simulink library "csc_ln200_lib_a"  (R2014b)
settings: Solver=ode45  SolverMode=SingleTasking  StartTime=0.0  StopTime=10.0  RelTol=1e-3
undefined symbols (not defined in the file or in its folder): est_time_step, sim_time_step_size
libraries: simulink x3, util_common_lib x2, csc_ln200_lib_a x2, util_info_lib x1, csu_imk_imu_kinematics_lib_a x1, csu_lnh_ln200_hardware_lib_a x1
settings Model: Creator=hcannon  LastModifiedBy=mstewart

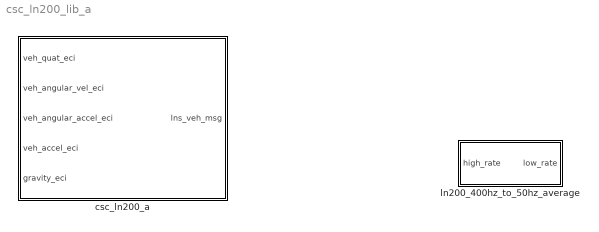
== system csc_ln200_lib_a ==
  csc_ln200_a : Subsystem
  ln200_400hz_to_50hz_average : Subsystem

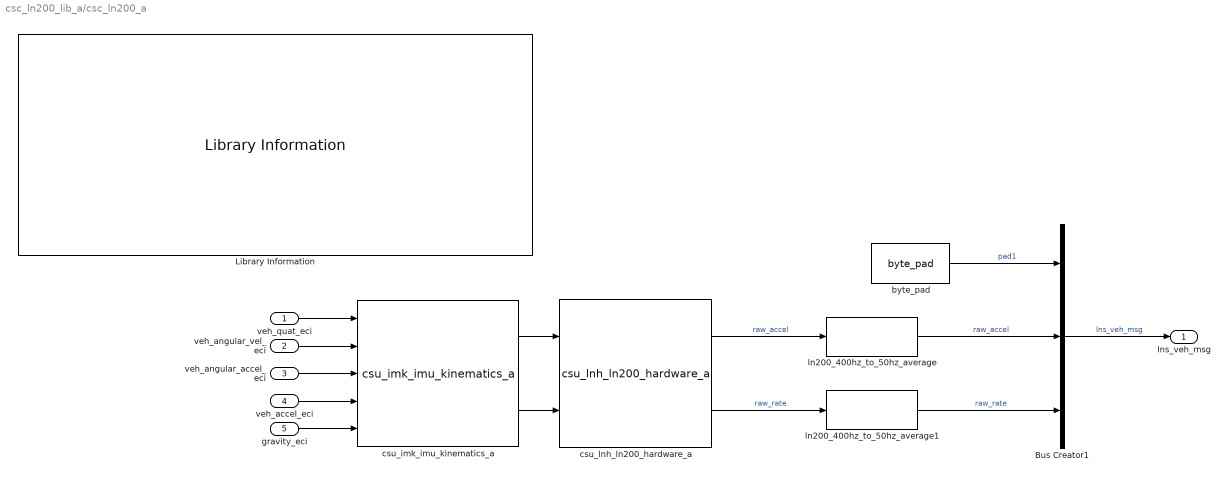
== system csc_ln200_lib_a/csc_ln200_a ==
  veh_quat_eci : Inport
  veh_angular_vel_eci : Inport  Port=2
  veh_angular_accel_eci : Inport  Port=3
  veh_accel_eci : Inport  Port=4
  gravity_eci : Inport  Port=5
  Bus Creator1 : BusCreator  Inputs=3  OutDataTypeStr=Bus: lns_veh_msg  NonVirtualBus=on
  Library Information : util_info_lib/Library Information  owner='NONE'
  byte_pad : util_common_lib/byte_pad  n_bytes=4
  csu_imk_imu_kinematics_a : csu_imk_imu_kinematics_lib_a/csu_imk_imu_kinematics_a
  csu_lnh_ln200_hardware_a : csu_lnh_ln200_hardware_lib_a/csu_lnh_ln200_hardware_a
  ln200_400hz_to_50hz_average : csc_ln200_lib_a/ln200_400hz_to_50hz_average
  ln200_400hz_to_50hz_average1 : csc_ln200_lib_a/ln200_400hz_to_50hz_average
  lns_veh_msg : Outport
  wires:
  byte_pad/1 -> Bus Creator1/1  "pad1"
  csu_lnh_ln200_hardware_a/2 -> ln200_400hz_to_50hz_average1/1  "raw_rate"
  csu_lnh_ln200_hardware_a/1 -> ln200_400hz_to_50hz_average/1  "raw_accel"
  csu_imk_imu_kinematics_a/1 -> csu_lnh_ln200_hardware_a/1
  csu_imk_imu_kinematics_a/2 -> csu_lnh_ln200_hardware_a/2
  Bus Creator1/1 -> lns_veh_msg/1  "lns_veh_msg"
  veh_quat_eci/1 -> csu_imk_imu_kinematics_a/1
  veh_angular_vel_eci/1 -> csu_imk_imu_kinematics_a/2
  veh_angular_accel_eci/1 -> csu_imk_imu_kinematics_a/3
  veh_accel_eci/1 -> csu_imk_imu_kinematics_a/4
  gravity_eci/1 -> csu_imk_imu_kinematics_a/5
  ln200_400hz_to_50hz_average/1 -> Bus Creator1/2  "raw_accel"
  ln200_400hz_to_50hz_average1/1 -> Bus Creator1/3  "raw_rate"

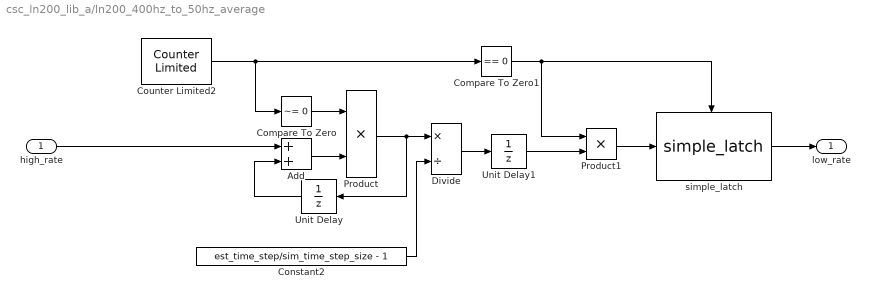
== system csc_ln200_lib_a/ln200_400hz_to_50hz_average ==
  high_rate : Inport
  Add : Sum
  Compare To Zero : simulink/Logic and Bit Operations/Compare To Zero  relop=~=  OutDataTypeStr=uint8
  Compare To Zero1 : simulink/Logic and Bit Operations/Compare To Zero  relop===  OutDataTypeStr=uint8
  Constant2 : Constant  Value=est_time_step/sim_time_step_size - 1
  Counter Limited2 : simulink/Sources/Counter Limited  uplimit=est_time_step/sim_time_step_size - 1  tsamp=-1
  Divide : Product  Inputs=*/
  Product : Product  RndMeth=Zero
  Product1 : Product  RndMeth=Zero
  Unit Delay : UnitDelay  SampleTime=-1
  Unit Delay1 : UnitDelay  SampleTime=-1
  simple_latch : util_common_lib/simple_latch  SystemSampleTime=-1
  low_rate : Outport
  wires:
  high_rate/1 -> Add/1
  Constant2/1 -> Divide/2
  Product/1 -> Unit Delay/1, Divide/1
  Unit Delay/1 -> Add/2
  Add/1 -> Product/2
  Compare To Zero/1 -> Product/1
  Divide/1 -> Unit Delay1/1
  Compare To Zero1/1 -> simple_latch/Trigger, Product1/1
  Counter Limited2/1 -> Compare To Zero/1, Compare To Zero1/1
  Unit Delay1/1 -> Product1/2
  Product1/1 -> simple_latch/1
  simple_latch/1 -> low_rate/1
